simulink model "system_simulation"  (R2019a)
settings: Solver=VariableStepAuto  StartTime=0.0  StopTime=10.0  RelTol=1e-3
settings Model: Creator=COMPUMARTS  LastModifiedBy=COMPUMARTS
settings OptimizationCC: DefaultParameterBehavior=Inlined  UseDivisionForNetSlopeComputation=on  GainParamInheritBuiltInType=on  UseFloatMulNetSlope=on  InlineInvariantSignals=on  PassReuseOutputArgsAs=Individual arguments  ZeroExternalMemoryAtStartup=off  ZeroInternalMemoryAtStartup=off  NoFixptDivByZeroProtection=on  EfficientFloat2IntCast=on  LifeSpan=1  OptimizeBlockOrder=speed  DifferentSizesBufferReuse=on
settings DebuggingCC: ParameterTunabilityLossMsg=error
settings HardwareCC: ProdLongLongMode=on
settings SFSimCC: MATLABDynamicMemAlloc=off
settings RTWCC: SystemTargetFile=ert.tlc  TemplateMakefile=ert_default_tmf  GenerateReport=on  IncludeHyperlinkInReport=on  LaunchReport=on  GenerateTraceInfo=on  GenerateTraceReport=on  GenerateTraceReportSl=on  GenerateTraceReportSf=on  GenerateTraceReportEml=on  GenerateCodeMetricsReport=on
settings CodeAppCC: ForceParamTrailComments=on  IgnoreCustomStorageClasses=off  OperatorAnnotations=on  SimulinkDataObjDesc=on  SFDataObjDesc=on  CustomSymbolStrGlobalVar=rt$N$M  CustomSymbolStrType=$N$M  CustomSymbolStrFcn=$N$M$F  CustomSymbolStrMacro=$N$M  InsertBlockDesc=on
settings ERTTargetCC: TargetLangStandard=C99 (ISO)  GenerateSampleERTMain=on  IncludeMdlTerminateFcn=off  CombineSignalStateStructs=on  SupportAbsoluteTime=off  SupportComplex=off  SupportContinuousTime=on  SupportNonInlinedSFcns=on  InlinedParameterPlacement=NonHierarchical  ERTCustomFileTemplate=example_file_process.tlc  ERTFilePackagingFormat=CompactWithDataFile

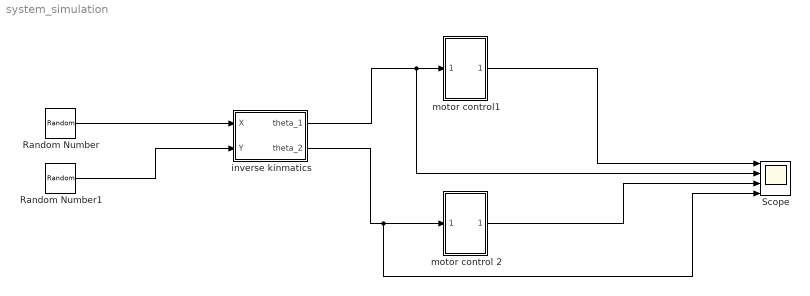
== system system_simulation ==
  Random Number : RandomNumber  SampleTime=0.1
  Random Number1 : RandomNumber  SampleTime=0.1
  Scope : Scope  NumInputPorts=4
  inverse kinmatics : MATLAB Function  TreatAsAtomicUnit=on
  motor control 2 : Subsystem
  "motor control1 " : Subsystem
  wires:
  inverse kinmatics/2(theta_2) -> Scope/4, motor control 2/1(In1)
  "motor control1 "/1(Out1) -> Scope/1
  Random Number/1 -> inverse kinmatics/1(X)
  Random Number1/1 -> inverse kinmatics/2(Y)
  inverse kinmatics/1(theta_1) -> Scope/2, "motor control1 "/1(In1)
  motor control 2/1(Out1) -> Scope/3

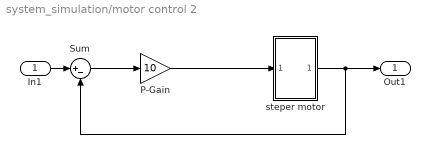
== system system_simulation/motor control 2 ==
  In1 : Inport
  P-Gain : Gain  Gain=10
  Sum : Sum  Inputs=|+-
  steper motor : Subsystem
  Out1 : Outport
  wires:
  P-Gain/1 -> steper motor/1(In1)
  Sum/1 -> P-Gain/1
  steper motor/1(Out1) -> Out1/1, Sum/2
  In1/1 -> Sum/1

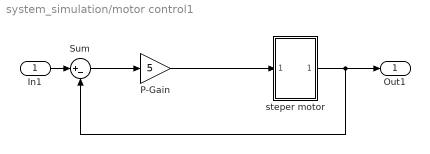
== system system_simulation/motor control1  ==
  In1 : Inport
  P-Gain : Gain  Gain=5
  Sum : Sum  Inputs=|+-
  steper motor : Subsystem
  Out1 : Outport
  wires:
  P-Gain/1 -> steper motor/1(In1)
  Sum/1 -> P-Gain/1
  steper motor/1(Out1) -> Out1/1, Sum/2
  In1/1 -> Sum/1

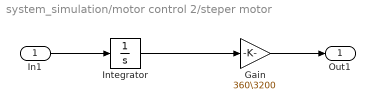
== system system_simulation/motor control 2/steper motor ==
  In1 : Inport
  Gain : Gain  Gain=360\3200
  Integrator : Integrator
  Out1 : Outport
  wires:
  Integrator/1 -> Gain/1
  In1/1 -> Integrator/1
  Gain/1 -> Out1/1

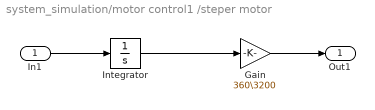
== system system_simulation/motor control1 /steper motor ==
  In1 : Inport
  Gain : Gain  Gain=360\3200
  Integrator : Integrator
  Out1 : Outport
  wires:
  Integrator/1 -> Gain/1
  In1/1 -> Integrator/1
  Gain/1 -> Out1/1

== matlab function system_simulation/inverse kinmatics ==
  data: X input; theta_1 output; Y input; theta_2 output

function [theta_1,theta_2] = fcn(X, Y)

    lenth = 0.25;
    lenth_6 = 0.2;
    theta_1=0;
    theta_2=0;
    val=50;
    val_2=50;
    
    
    X=X/100;
    Y=Y/100;
    K1 = sqrt(((X+(lenth_6/2))^2)+(Y^2));
    K2 = sqrt(((X-(lenth_6/2))^2)+(Y^2));
    
    if K1 ~= 0
        if K2 ~=0 
            val= ((K1^2)/(2*lenth*K1));
            val_2= ((K2^2)/(2*lenth*K2));
        end
    end
    if(val < 1)
        if (val > -1)
            if (val_2<1)
                if (val_2>-1)
                    pthai_1 = acos((K1^2)/(2*lenth*K1));
                    pthai_2 = acos((K2^2)/(2*lenth*K2));
    
                    zeta_1 = atan2(Y,(X+(lenth_6/2)));
                    zeta_2 = atan2(Y,(X-(lenth_6/2)));
    
                    theta_1 = rad2deg(zeta_1 + pthai_1);  
                    theta_2 = rad2deg(zeta_2 - pthai_2);
                   
                end
            end
        end
    end
